simulink model "algorithms_SEPIC"  (R2015b)
settings: Solver=VariableStepAuto  StartTime=0.0  StopTime=2  RelTol=1e-3
libraries: powerlib x55, re_lib x5, simulink x4, powerlib_meascontrol x1
settings Model: Creator=SPIRO-POWER  LastModifiedBy=SPIRO-POWER
settings SolverCC: AlgebraicLoopSolver=LineSearch

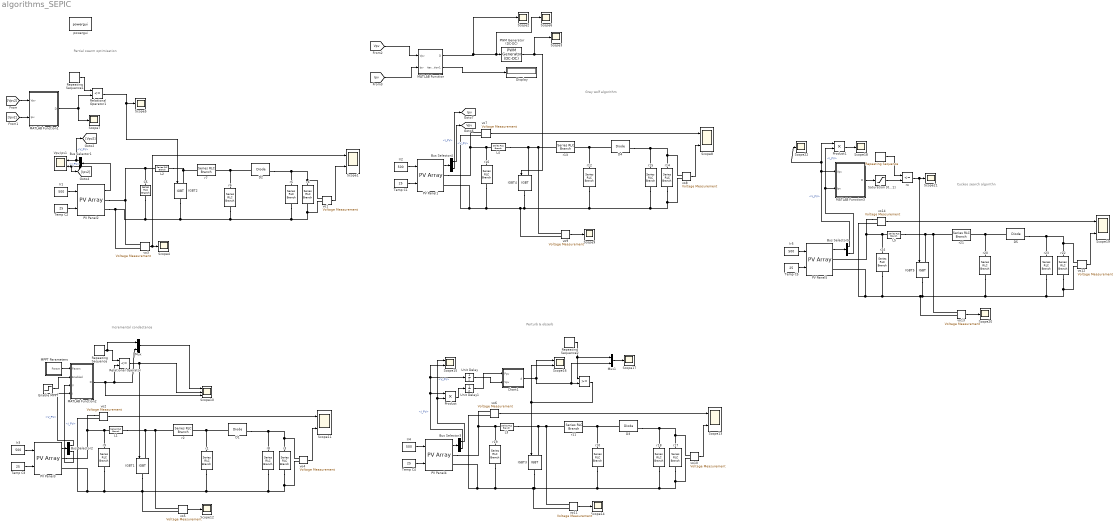
== system algorithms_SEPIC ==
  note: Cuckoo search algorithn
  note: Perturb & obserb
  note: Incremental condactance
  note: Grey wolf algorithm
  note: Partial swarm optimisation
  "   " : simulink/Sources/Repeating Sequence  rep_seq_t=[0 0.001]  rep_seq_y=[0 1]
  "    " : RelationalOperator  OutDataTypeStr=boolean
  Bus Selector{1..5} (5 alike) : BusSelector  OutputSignals=V_PV,I_PV
  C5 : powerlib/Elements/Series RLC Branch  LConnTagsString=__new0  RConnTagsString=__new0  BranchType=C  Resistance=1.0  Inductance=1.0  SetiL0=off  InitialCurrent=0  Capacitance=200e-6  Setx0=off  InitialVoltage=0  Measurements=Branch voltage
  Chart1 : Stateflow chart  TreatAsAtomicUnit=on
  D{1..5} (5 alike) : powerlib/Power Electronics/Diode  Ron=0.001  Lon=0  Vf=0.8  IC=0  UseSnubber=off  Rs=500  Cs=250e-9  Measurements=on
  Display : Display
  Enable MPPT : Step  Time=0.3  SampleTime=0
  IGBT{1..5} (5 alike) : powerlib/Power Electronics/IGBT  Ron=0.001  Lon=0  Vf=0  Tf=0  Tt=0  IC=0  Rs=1e5  Cs=inf  Measurements=off
  Ir{1..5} (5 alike) : Constant  Value=500
  L{1..5} (5 alike) : powerlib/Elements/Series RLC Branch  LConnTagsString=__new0  RConnTagsString=__new0  BranchType=L  Resistance=0.005  Inductance=5e-3  SetiL0=off  InitialCurrent=0  Capacitance=1e-6  Setx0=off  InitialVoltage=0  Measurements=None
  MATLAB Function : MATLAB Function  TreatAsAtomicUnit=on
  MATLAB Function1 : MATLAB Function  TreatAsAtomicUnit=on
  MATLAB Function2 : MATLAB Function  TreatAsAtomicUnit=on
  MATLAB Function3 : MATLAB Function  TreatAsAtomicUnit=on
  MPPT Parameters : Subsystem
  Mux : Mux  Inputs=2
  Mux1 : Mux  Inputs=2
  PV Panel{1..5} (5 alike) : re_lib/Solar/PV Array  Npar=1  Nser=1  PlotType=one module @ 25 deg.C & specified irradiances  S_vec=1000  Temp_C_vec="[ 45 25  ]"  ModuleName=User-defined  PlotWhenSelected=off  Pm=59.85  Ncell=36  Voc=21.1  Isc=3.8  Vm=17.1  Im=3.5  beta_Voc_pc=-0.38  alpha_Isc_pc=0.065  beta_Voc=-0.08018  alpha_Isc=0.00247  IL=3.8128  I0=2.5245e-10  nI=0.97484  Rsh=153.5644  Rs=0.38572  BAL=off  Tc=1e-6  Tfilter=0.0001
      settings: AttributesFormatString=|
      | %<ModuleName>
      | %<Nser>-module string
      | %<Npar> parallel strings
  PWM Generator (DC-DC) : powerlib_meascontrol/Pulse & Signal Generators/PWM Generator (DC-DC)  Fsw=1000  Ts=0
  Product : Product
  Product1 : Product
  Relational Operator : RelationalOperator  Operator=<=  OutDataTypeStr=boolean
  Relational Operator1 : RelationalOperator  Operator=<=  OutDataTypeStr=boolean
  Repeating Sequence : simulink/Sources/Repeating Sequence  rep_seq_t=[0 0.001]  rep_seq_y=[0 1]
  Repeating Sequence1 : simulink/Sources/Repeating Sequence  rep_seq_t=[0 0.001]  rep_seq_y=[0 1]
  Repeating Sequence2 : simulink/Sources/Repeating Sequence  rep_seq_t=[0 0.001]  rep_seq_y=[0 1]
  Saturation [0...1] : Saturate  UpperLimit=0.8  LowerLimit=0
  Scope{1,8,11,13,15..16,19} (7 alike) : Scope  NumInputPorts=2
  Scope10 : Scope  NumInputPorts=3
  Scope{2..7,9,12,14,17..18,20..22} (14 alike) : Scope
  Temp C{1..5} (5 alike) : Constant  Value=25
  Unit Delay : UnitDelay
  Unit Delay1 : UnitDelay
  Vpv,Ipv1 : Scope  NumInputPorts=2
  powergui : powerlib/powergui  Priority=1  SimulationMode=Discrete  SolverType=Tustin/Backward Euler (TBE)  SampleTime=50e-6  frequency=60  SPID=off  DisableSnubberDevices=off  DisableRonSwitches=off  DisableVfSwitches=off  SwTol=0  DisplayEquations=off  Interpol=off  ExternalGateDelay=off  methode=off  Ts=10  FunctionMessages=off  echomessages=off  HookPort=off  EnableUseOfTLC=off  x0status=blocks  frequencyindice=0  Pbase=100e6  ErrMax=1e-4  Iterations=50  UnitsV=kV  UnitsW=MW  buscounter=0  RestoreLinks=warning  ResistiveCurrentMeasurement=off  Frange=[0:2:500]  Ylog=off  Xlog=on  ShowGrid=off  save=off  variable=ZData  structure=0  ZoomFFT=off  StartTime=0.0  cycles=1  DisplayStyle=1  fundamental=60  FreqAxis=off  MaxFrequency=1000  frequencyindicesteady=1  RmsSteady=1  display=off
  r{1,6,10,12,20} (5 alike) : powerlib/Elements/Series RLC Branch  LConnTagsString=__new0  RConnTagsString=__new0  BranchType=L  Resistance=1  Inductance=15e-3  SetiL0=off  InitialCurrent=0  Capacitance=1000e-6  Setx0=off  InitialVoltage=0  Measurements=None
  r{2,7,11,13,21} (5 alike) : powerlib/Elements/Series RLC Branch  LConnTagsString=__new0  RConnTagsString=__new0  BranchType=C  Resistance=1  Inductance=1e-3  SetiL0=off  InitialCurrent=0  Capacitance=1000e-6  Setx0=off  InitialVoltage=0  Measurements=None
  r{3,14,17,22} (4 alike) : powerlib/Elements/Series RLC Branch  LConnTagsString=__new0  RConnTagsString=__new0  BranchType=R  Resistance=100  Inductance=1e-3  SetiL0=off  InitialCurrent=0  Capacitance=100e-6  Setx0=off  InitialVoltage=0  Measurements=None
  r{5,8,15,18,23} (5 alike) : powerlib/Elements/Series RLC Branch  LConnTagsString=__new0  RConnTagsString=__new0  BranchType=C  Resistance=1  Inductance=1e-3  SetiL0=off  InitialCurrent=0  Capacitance=2000e-6  Setx0=off  InitialVoltage=0  Measurements=None
  r{9,16,19,24} (4 alike) : powerlib/Elements/Series RLC Branch  LConnTagsString=__new0  RConnTagsString=__new0  BranchType=C  Resistance=1  Inductance=1e-3  SetiL0=off  InitialCurrent=0  Capacitance=200e-6  Setx0=off  InitialVoltage=0  Measurements=None
  r4 : powerlib/Elements/Series RLC Branch  LConnTagsString=__new0  RConnTagsString=__new0  BranchType=R  Resistance=100  Inductance=1e-3  SetiL0=off  InitialCurrent=0  Capacitance=1e-6  Setx0=off  InitialVoltage=0  Measurements=None
  ro : RelationalOperator  Operator=<=  OutDataTypeStr=boolean
  vo{1..14} (14 alike) : powerlib/Measurements/Voltage Measurement  PhasorSimulation=off  OutputType=Complex  PSBequivalent=0
  tag scope: Ipv=global, Vpv=global
  wires:
  PV Panel2/1 -> Bus Selector1/1
  Relational Operator1/1 -> IGBT2/1, Scope5/1
  Bus Selector1/1 -> Vpv,Ipv1/1, [Vpv2]  "<V_PV>"
  Bus Selector1/2 -> [Ipv2], Vpv,Ipv1/2  "<I_PV>"
  vo3/1 -> Scope1/1, Scope4/1
  Repeating Sequence1/1 -> Relational Operator1/1
  [Vpv2] -> MATLAB Function1/1(Vpv)
  [Ipv2] -> MATLAB Function1/2(Ipv)
  vo1/1 -> Scope1/2
  vo7/1 -> Scope8/1
  vo8/1 -> Scope8/2
  Ir2/1 -> PV Panel1/1
  Temp C1/1 -> PV Panel1/2
  PV Panel1/1 -> Bus Selector4/1
  Bus Selector4/1 -> [Vpv]  "<V_PV>"
  Bus Selector4/2 -> [Ipv]  "<I_PV>"
  PWM Generator (DC-DC)/1 -> IGBT4/1, Scope3/1
  MATLAB Function/2(iteration1) -> Display/1
  [Vpv] -> MATLAB Function/1(Vpv)
  [Ipv] -> MATLAB Function/2(Ipv)
  MATLAB Function/1(D) -> Scope6/1, PWM Generator (DC-DC)/1, Scope2/1
  MATLAB Function1/1(D) -> Scope7/1, Relational Operator1/2
  Ir1/1 -> PV Panel2/1
  Temp C2/1 -> PV Panel2/2
  vo9/1 -> Scope9/1
  Enable MPPT/1 -> MATLAB Function2/2(Enabled)
  MPPT Parameters/1(Param) -> MATLAB Function2/1(Param)
  Repeating Sequence/1 -> Mux/1, Relational Operator/1
  MATLAB Function2/1(D) -> Scope10/3, Mux/2, Relational Operator/2
  Mux/1 -> Scope10/1
  vo2/1 -> Scope11/1
  vo4/1 -> Scope11/2
  Ir3/1 -> PV Panel3/1
  Temp C3/1 -> PV Panel3/2
  PV Panel3/1 -> Bus Selector2/1
  Bus Selector2/1 -> MATLAB Function2/4(I)  "<V_PV>"
  Bus Selector2/2 -> MATLAB Function2/3(V)  "<I_PV>"
  vo5/1 -> Scope12/1
  Relational Operator/1 -> Scope10/2, IGBT1/1
  vo6/1 -> Scope13/1
  vo10/1 -> Scope13/2
  Ir4/1 -> PV Panel4/1
  Temp C4/1 -> PV Panel4/2
  PV Panel4/1 -> Bus Selector3/1
  vo11/1 -> Scope14/1
  Bus Selector3/1 -> Product/2, Scope15/1  "<V_PV>"
  Bus Selector3/2 -> Product/1, Unit Delay/1, Scope15/2  "<I_PV>"
  "    "/1 -> IGBT3/1, Scope16/2
  Chart1/1(d) -> Scope16/1, Mux1/2, "    "/2
  Product/1 -> Unit Delay1/1
  Unit Delay/1 -> Chart1/2(Vpv)
  Unit Delay1/1 -> Chart1/1(Ppv)
  Repeating Sequence2/1 -> Mux1/1, "    "/1
  Mux1/1 -> Scope17/1
  ro/1 -> Scope21/1, IGBT5/1
  Bus Selector5/2 -> MATLAB Function3/2(Ipv), Product1/2  "<I_PV>"
  MATLAB Function3/1(D) -> Saturation [0...1]/1
  Saturation [0...1]/1 -> ro/2
  Bus Selector5/1 -> Product1/1, Scope22/1, MATLAB Function3/1(Vpv)  "<V_PV>"
  Product1/1 -> Scope18/1
  "   "/1 -> ro/1
  vo14/1 -> Scope19/1
  vo12/1 -> Scope19/2
  vo13/1 -> Scope20/1
  Ir5/1 -> PV Panel5/1
  Temp C5/1 -> PV Panel5/2
  PV Panel5/1 -> Bus Selector5/1
  connections:
  L2/RConn1 -- r7/LConn1 -- IGBT2/LConn1
  vo3/LConn1 -- PV Panel2/RConn1 -- C5/LConn1 -- L2/LConn1
  D2/LConn1 -- r6/RConn1 -- r7/RConn1
  r5/LConn1 -- vo1/LConn1 -- r4/LConn1 -- D2/RConn1
  IGBT2/RConn1 -- r6/LConn1 -- r5/RConn1 -- vo1/LConn2 -- r4/RConn1 -- C5/RConn1 -- PV Panel2/RConn2 -- vo3/LConn2
  D4/LConn1 -- r12/RConn1 -- r13/RConn1
  vo8/LConn1 -- r14/LConn1 -- D4/RConn1 -- r15/LConn1
  vo8/LConn2 -- r14/RConn1 -- r15/RConn1 -- r12/LConn1 -- vo9/LConn2 -- r16/RConn1 -- vo7/LConn2 -- PV Panel1/RConn2 -- IGBT4/RConn1
  L4/RConn1 -- vo9/LConn1 -- r13/LConn1 -- IGBT4/LConn1
  L4/LConn1 -- r16/LConn1 -- PV Panel1/RConn1 -- vo7/LConn1
  D1/LConn1 -- r1/RConn1 -- r2/RConn1
  r8/LConn1 -- r3/LConn1 -- vo4/LConn1 -- D1/RConn1
  vo4/LConn2 -- r3/RConn1 -- r8/RConn1 -- r1/LConn1 -- r9/RConn1 -- vo2/LConn2 -- PV Panel3/RConn2 -- vo5/LConn2 -- IGBT1/RConn1
  L1/RConn1 -- vo5/LConn1 -- r2/LConn1 -- IGBT1/LConn1
  vo2/LConn1 -- PV Panel3/RConn1 -- r9/LConn1 -- L1/LConn1
  r10/RConn1 -- D3/LConn1 -- r11/RConn1
  r17/LConn1 -- r18/LConn1 -- D3/RConn1 -- vo10/LConn1
  r17/RConn1 -- vo11/LConn2 -- PV Panel4/RConn2 -- vo6/LConn2 -- r19/RConn1 -- IGBT3/RConn1 -- r10/LConn1 -- r18/RConn1 -- vo10/LConn2
  vo11/LConn1 -- L3/RConn1 -- IGBT3/LConn1 -- r11/LConn1
  PV Panel4/RConn1 -- L3/LConn1 -- r19/LConn1 -- vo6/LConn1
  r20/RConn1 -- D5/LConn1 -- r21/RConn1
  r22/LConn1 -- vo12/LConn1 -- r23/LConn1 -- D5/RConn1
  vo13/LConn2 -- IGBT5/RConn1 -- r20/LConn1 -- r23/RConn1 -- vo12/LConn2 -- r22/RConn1 -- r24/RConn1 -- PV Panel5/RConn2 -- vo14/LConn2
  vo13/LConn1 -- L5/RConn1 -- IGBT5/LConn1 -- r21/LConn1
  vo14/LConn1 -- PV Panel5/RConn1 -- L5/LConn1 -- r24/LConn1

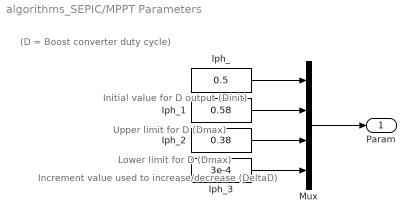
== system algorithms_SEPIC/MPPT Parameters ==
  note: Upper limit for D (Dmax)
  note: Increment value used to increase/decrease (DeltaD)
  note: Initial value for D output (Dinit)
  note: (D = Boost converter duty cycle)
  note: Lower limit for D (Dmax)
  Iph_ : Constant  Value=0.5
  Iph_1 : Constant  Value=0.58
  Iph_2 : Constant  Value=0.38
  Iph_3 : Constant  Value=3e-4
  Mux : Mux
  Param : Outport
  wires:
  Iph_/1 -> Mux/1
  Iph_1/1 -> Mux/2
  Iph_2/1 -> Mux/3
  Iph_3/1 -> Mux/4
  Mux/1 -> Param/1

== matlab function algorithms_SEPIC/MATLAB Function1 ==
  settings: updateMethod=DISCRETE  sampleTime=1e-4
  data: Vpv input; D output; Ipv input
function D = PSO(Vpv,Ipv)
%#codegen
persistent u;
persistent dcurrent;
persistent pbest;
persistent p;
persistent dc;
persistent v;
persistent counter;
persistent gbest;
if(isempty(counter))
    counter=0;
end
if(isempty(dcurrent))
    dcurrent=0.5;
end
if(isempty(gbest))
    gbest=0.5;
end
if(isempty(p))
    p=zeros(4,1);
end

if(isempty(v))
    v=zeros(4,1);
end

if(isempty(pbest))
    pbest=zeros(4,1);
end
if(isempty(u))
    u=0;
end
if(isempty(dc))
    dc=zeros(4,1);
    dc(1)=0;
    dc(2)=0.3;
    dc(3)=0.5;
    dc(4)=0.9;
end
if(counter>=1 && counter<300)
    D=dcurrent;
    counter=counter+1;
    return;
end
counter=0;

if(u>=1 && u<=4)
    if((Vpv*Ipv)>p(u))
        p(u)=Vpv*Ipv;
        pbest(u)=dcurrent;
    end
end
u=u+1;
if(u==6)
    u=1;
end
if(u==1)
    D=dc(u);
    dcurrent=D;
    counter=1;
    return;
elseif(u==2)
    D=dc(u);
    dcurrent=D;
    counter=1;
    return;
elseif(u==3)
    D=dc(u);
    dcurrent=D;
    counter=1;
    return;
elseif(u==4)
    D=dc(u);
    dcurrent=D;
    counter=1;
    return;
elseif(u==5 )
    [m,i]=max(p);
    gbest=pbest(i);
    D=gbest;
    dcurrent=D;
    counter=1;
    %update velocity and duty cycle
    v(1)=updatevelocity(v(1),pbest(1),dc(1),gbest)
    v(2)=updatevelocity(v(2),pbest(2),dc(2),gbest)
    v(3)=updatevelocity(v(3),pbest(3),dc(3),gbest)
    v(4)=updatevelocity(v(4),pbest(4),dc(4),gbest)
    %update duty cycle
    dc(1)=updateduty(dc(1),v(1))
    dc(2)=updateduty(dc(2),v(2))
    dc(3)=updateduty(dc(3),v(3))
    dc(4)=updateduty(dc(4),v(4))
    
    return;
    
else
    u
    y='hello'
    D=0.1
    
end


end
function vfinal=updatevelocity(velocity,pobest,d,gwbest)
% PSO Parameters
w=0.4;
%w=(1.1-(pobest/gwbest));            % Inertia Weight
             % Inertia Weight Damping Ratio
c1=1.2;         % Personal Learning Coefficient
c2=2;         % Global Learning Coefficient

% If you would like to use Constriction Coefficients for PSO,
% uncomment the following block and comment the above set of parameters.

% % Constriction Coefficients
% phi1=2.05;
% phi2=2.05;
% phi=phi1+phi2;
% chi=2/(phi-2+sqrt(phi^2-4*phi));
% w=chi;          % Inertia Weight
% wdamp=1;        % Inertia Weight Damping Ratio
% c1=chi*phi1;    % Personal Learning Coefficient
% c2=chi*phi2;    % Global Learning Coefficient
vfinal = (w*velocity)+(c1*rand(1)*(pobest-d))+(c2*rand(1)*(gwbest-d));
end
function dfinal=updateduty(d,velocity)
dup=d+velocity;
if(dup>1)
    dfinal=1;
elseif(dup<0)
    dfinal=0;
else
    dfinal=dup;
end
end

== matlab function algorithms_SEPIC/MATLAB Function2 ==
  data: Param input; D output; Enabled input; V input; I input
function D  = InCon(Param, Enabled, V, I)

% MPPT controller based on the IncrementalConductance algorithm.
% D output = Duty cycle of the boost converter (value between 0 and 1)
%
% Enabled input = 1 to enable the MPPT controller
% V input = PV array terminal voltage (V)
% I input = PV array current (A)
%
% Param input:
Dinit = Param(1);  %Initial value for D output
Dmax = Param(2);   %Maximum value for D
Dmin = Param(3);   %Minimum value for D
deltaD = Param(4); %Increment value used to increase/decrease the duty cycle D
% ( increasing D = decreasing Vref )
%
% Define constants
E = 0.002; % Maximum dI/dV error

persistent Vold Iold Dold ;

dataType = 'double';

if isempty(Vold)
    Vold=0;
    Iold=0;
    Dold=Dinit;
end
dV= V - Vold;
dI= I - Iold;

 if dV == 0 & Enabled ~=0
     if dI == 0
         D=Dold; % No change
     elseif dI > 0
        D = Dold - deltaD; % Increase Vref
     else
         D = Dold + deltaD; % Decrease Vref
     end
 else
    if abs(dI/dV + I/V) <= E
       D=Dold; % No change
    else
      if dI/dV > -I/V + E
         D = Dold - deltaD; % Increase Vref
      else
         D = Dold + deltaD; % Decrease Vref
      end
    end
 end
 
if D >= Dmax | D<= Dmin
    D=Dold;
end

Dold=D;
Vold=V;
Iold=I;

== matlab function algorithms_SEPIC/MATLAB Function ==
  data: Vpv input; D output; Ipv input; iteration1 output
function [D,iteration1] = GWO(Vpv,Ipv)
dim = 1;
m = 5;
persistent dc
persistent fitness
persistent D_new;
persistent alpha;
persistent alpha_pos Beta_pos ;
persistent iteration Beta_score Delta_score Delta_pos;
persistent Gmax;
persistent i
persistent tol
if(isempty(iteration))
    iteration=0;
    tol=100;
end
if(isempty(D_new))
    D_new = 0.5;
end
% if(isempty(Gbest))
%     Gbest = 0.5;
% end
if(isempty(Gmax))
    Gmax=0;
end
if(isempty(alpha))
    alpha=0;
end
if (isempty(Beta_pos))
    alpha_pos=zeros(1,dim);
    Beta_pos=zeros(1,dim);
    Delta_pos=zeros(1,dim);
    Beta_score=0;
    Delta_score=0;
end
if(isempty(alpha))
    alpha=0;
end
if (isempty(alpha_pos))
    alpha_pos=zeros(1,dim);
end

if(isempty(dc))
    dc=zeros(5,1);
    
    dc(1)=0.1;
    dc(2)=0.2;
    dc(3)=0.3;
    dc(4)=0.4;
    dc(5)=0.5;
%     dc(6)=0.6;
%     dc(7)=0.7;
%     dc(8)=0.8;
%     dc(9)=0.9;
%     dc(10)=1;
end
if (isempty(i))
    i=0;
    D = 0.5;
end
% D = 0.5;
iteration1 = 0;
if (iteration <100 )
        iteration1=iteration;
        
    if i<5
        i = i+1;
        Flag4ub=dc(i,:)>1;
        Flag4lb=dc(i,:)<0;
        dc(i)=(dc(i).*(~(Flag4ub+Flag4lb)))+1.*Flag4ub;               
        
        fitness=Vpv*Ipv;
        tol = abs(alpha-fitness);
        if fitness>alpha 
            alpha=fitness; % Update alpha
            alpha_pos=dc(i);
        end
        if fitness<alpha && fitness>Beta_score 
            Beta_score=fitness; % Update beta
            Beta_pos=dc(i);
        end
        
        if fitness<alpha && fitness<Beta_score && fitness>Delta_score 
            Delta_score=fitness; % Update delta
            Delta_pos=dc(i);
        end
        D_new =dc(i);
        D = dc(i);
        return;
        
    end
    iteration = iteration+1;
    i = 0;
end
D = alpha_pos;
end

== stateflow chart algorithms_SEPIC/Chart1 ==
  state input1
    entry:Pprev=40;
    Vprev=20;
    d=0.5
  state calc_
    entry:dP=Ppv-Pprev;
    dV=Vpv-Vprev;
  state invrese
    entry:
    d=d+0.01;
  state decrese
    entry:
    d=d-0.01;
  state decrese1
    entry:
    d=d+0.01;
  state decrese2
    entry:
    d=d-0.01;
  state return
    entry:
    Pprev=Ppv;
    Vprev=Vpv;
  (default) -> input1
  input1 -> calc_
  return -> calc_
  calc_ -> (junction 15) [order 1] : [dP>0]
  calc_ -> (junction 24) [order 2] : [dP<0]
  (junction 24) -> decrese2 [order 2] : [dV>0]
  (junction 15) -> invrese [order 1] : [dV>0]
  (junction 15) -> decrese [order 2] : [dV<0]
  (junction 24) -> return [order 3]
  (junction 24) -> decrese1 [order 1] : [dV<0]
  (junction 15) -> return [order 3]
  invrese -> return
  decrese -> return
  decrese1 -> return
  decrese2 -> return
  data: Ppv input; Vpv input; d output; Pprev local; dP local; dV local; Vprev local

== matlab function algorithms_SEPIC/MATLAB Function3 ==
  settings: updateMethod=DISCRETE  sampleTime=1e-4
  data: Vpv input; D output; Ipv input
function D = Cuckoo(Vpv,Ipv)
%#codegen
persistent u;
persistent dcurrent;
persistent p;
persistent dc;
persistent dbest;
persistent counter;
persistent iworst;
persistent discover;
if(isempty(discover))
    discover=0;
end
if(isempty(counter))
    counter=0;
end
if(isempty(dcurrent))
    dcurrent=0.5;
end
if(isempty(iworst))
    iworst=0;
end



if(isempty(dbest))
    dbest=0;
end
if(isempty(p))
    p=zeros(4,1);
end
if(isempty(u))
    u=0;
end
if(isempty(dc))
    dc=zeros(4,1);
    dc(1)=0;
    dc(2)=0.3;
    dc(3)=0.5;
    dc(4)=0.9;
end
if(counter>=1 && counter<150)
    D=dcurrent;
    counter=counter+1;
    return;
end
counter=0;

if(u>=1 && u<=4)
    p(u)=Vpv*Ipv;
end
u=u+1;
if(u==7)
    u=1;
end
if(u==1)
    D=dc(u);
    dcurrent=D;
    counter=1;
    return;
elseif(u==2)
    D=dc(u);
    dcurrent=D;
    counter=1;
    return;
elseif(u==3)
    D=dc(u);
    dcurrent=D;
    counter=1;
    return;
elseif(u==4)
    D=dc(u);
    dcurrent=D;
    counter=1;
    return;
elseif(u==5 || u==6 )
    if(u==5)
        if(rand(1)>0.25)
            discover=1;
            [m,i]=max(p)
            dbest=dc(i);
            %determine the worst nest
            [m,iworst]=min(p);
            %build new nest
            %dc(iworst)=dbest;
            dc(iworst)=levyflight(dbest,dc(iworst));
            %dc(iworst)=withinlimits(dc(iworst));
            D=dc(iworst);
            dcurrent=D;
            counter=1;
            return;
        else
            u=u+1;
            [m,i]=max(p)
            dbest=dc(i);
            D=dbest;
            dcurrent=D;
            counter=1;
            dc(1)=levyflight(dbest,dc(1))
            % dc(1)=withinlimits(dc(1))
            dc(2)=levyflight(dbest,dc(2))
            %dc(2)=withinlimits(dc(2))
            dc(3)=levyflight(dbest,dc(3))
            % dc(3)=withinlimits(dc(3))
            dc(4)=levyflight(dbest,dc(4))
            % dc(4)=withinlimits(dc(4))
            return;
        end
        
    else
        %calculate new power of new nest
        p(iworst)=Vpv*Ipv;
        %determine the best nest
        [m,i]=max(p);
        dbest=dc(i);
        D=dbest;
        dcurrent=D;
        counter=1;
        
        dc(1)=levyflight(dbest,dc(1))
        % dc(1)=withinlimits(dc(1))
        dc(2)=levyflight(dbest,dc(2))
        %dc(2)=withinlimits(dc(2))
        dc(3)=levyflight(dbest,dc(3))
        % dc(3)=withinlimits(dc(3))
        dc(4)=levyflight(dbest,dc(4))
        % dc(4)=withinlimits(dc(4))
        discover=0;
        return;
    end
    
else
    u
    y='hello'
    D=0.1
    
end


end
function dfinal=levyflight(dbest,d)
beta=3/2;
kcoeff=0.8;
sigmau=(gamma(1+beta)*sin(pi*beta/2)/(gamma((1+beta)/2)*beta*2^((beta-1)/2)))^(1/beta);
sigmav=1;
u=normrnd(0,(sigmau)^2);
v=normrnd(0,(sigmav)^2);
dup=d+(kcoeff*(abs(u)/((abs(v))^(1/beta)))*(dbest-d));


if(dup>1)
    dfinal=1;
elseif(dup<0)
    dfinal=0;
else
    dfinal=dup;
end
end
